simulink model "sara_restored_from_autosave"  (R2016a)
settings: Solver=VariableStepAuto  StartTime=0.0  StopTime=10  RelTol=1e-3
values from neighbouring files (symbols this model uses):
  s = a(1)*(t.^3)+a(2)*(t.^2)+a(3)*t+a(4)    [quydao.m]
undefined symbols (not defined in the file or in its folder): gia, k1, k2, k3, k4, RootGround, RootPart, sara
libraries: mblibv1 x17, simulink x1
settings Model: Creator=Admin  LastModifiedBy=Admin
settings GRTTargetCC: GeneratePreprocessorConditionals=Use local settings
settings SimMechanicsCC: VisOnUpdateDiagram=on  VisDuringSimulation=on

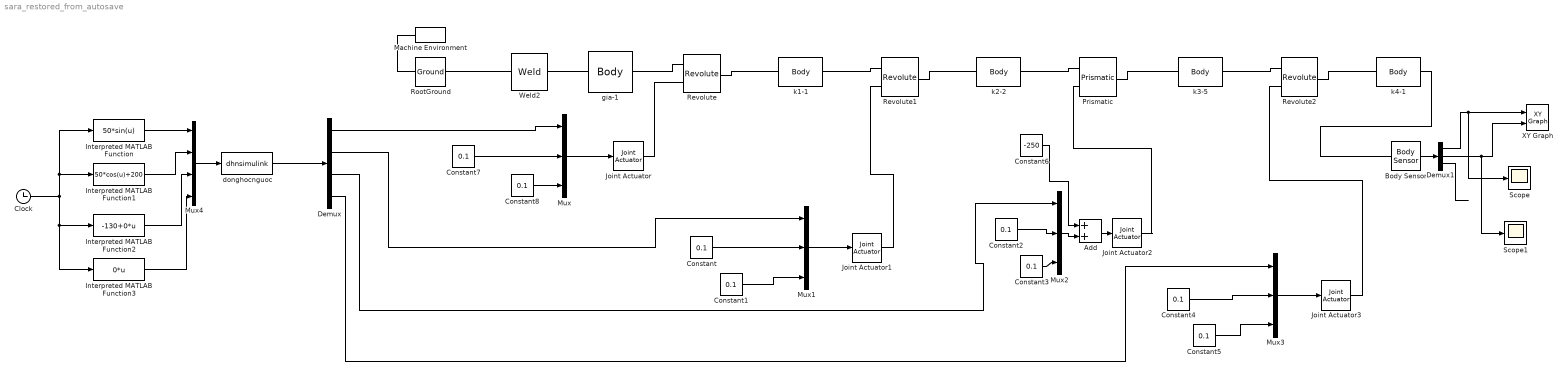
== system sara_restored_from_autosave ==
  Add : Sum
  Body Sensor : mblibv1/Sensors &  Actuators/Body Sensor  UpdateFromCAD=off  PhysicalDomain=Mechanical  PortType=blob  Muxed=on  Pose=off  Angle=on  AngleUnits=deg  ArcVelocity=off  ArcVelocityUnits=deg/s  ArcAcceleration=off  ArcAccelerationUnits=deg/s^2  CoordPosition=on  CoordPositionUnits=mm  Velocity=off  VelocityUnits=m/s  Acceleration=off  AccelerationUnits=m/s^2  Quaternion=on  QuaternionDT=off  QuaternionDDT=off  QuaternionUnits=off  OutputVector=[1]  ActiveIO=on  Width=3  DialogClass=MechanicalSensorBlock  ReferenceFrame=Absolute (World)
  Clock : Clock
  Constant{,1..5,7..8} (8 alike) : Constant  Value=0.1
  Constant6 : Constant  Value=-250
  Demux : Demux
  Demux1 : Demux  Outputs=3
  Interpreted MATLAB Function : MATLABFcn  MATLABFcn=50*sin(u)
  Interpreted MATLAB Function1 : MATLABFcn  MATLABFcn=50*cos(u)+200
  Interpreted MATLAB Function2 : MATLABFcn  MATLABFcn=-130+0*u
  Interpreted MATLAB Function3 : MATLABFcn  MATLABFcn=0*u
  Joint Actuator : mblibv1/Sensors &  Actuators/Joint Actuator  UpdateFromCAD=off  PhysicalDomain=Mechanical  PortType=blob  ActuationStyle=Motion  AngleUnits=rad  ArcVelocityUnits=rad/s  ArcAccelerationUnits=rad/s^2  CoordPositionUnits=m  VelocityUnits=m/s  AccelerationUnits=m/s^2  ForceUnits=N  TorqueUnits=N*m  ActiveIO=on  Width=3  DialogClass=MechanicalActuatorBlock  Primitive=R1  ReferenceFrame=Absolute (World)
  Joint Actuator1 : mblibv1/Sensors &  Actuators/Joint Actuator  UpdateFromCAD=off  PhysicalDomain=Mechanical  PortType=blob  ActuationStyle=Motion  AngleUnits=rad  ArcVelocityUnits=rad/s  ArcAccelerationUnits=rad/s^2  CoordPositionUnits=m  VelocityUnits=m/s  AccelerationUnits=m/s^2  ForceUnits=N  TorqueUnits=N*m  ActiveIO=on  Width=3  DialogClass=MechanicalActuatorBlock  Primitive=R1  ReferenceFrame=Absolute (World)
  Joint Actuator2 : mblibv1/Sensors &  Actuators/Joint Actuator  UpdateFromCAD=off  PhysicalDomain=Mechanical  PortType=blob  ActuationStyle=Motion  AngleUnits=deg  ArcVelocityUnits=deg/s  ArcAccelerationUnits=deg/s^2  CoordPositionUnits=mm  VelocityUnits=mm/s  AccelerationUnits=mm/s^2  ForceUnits=N  TorqueUnits=N*m  ActiveIO=on  Width=3  DialogClass=MechanicalActuatorBlock  Primitive=P1  ReferenceFrame=Absolute (World)
  Joint Actuator3 : mblibv1/Sensors &  Actuators/Joint Actuator  UpdateFromCAD=off  PhysicalDomain=Mechanical  PortType=blob  ActuationStyle=Motion  AngleUnits=rad  ArcVelocityUnits=rad/s  ArcAccelerationUnits=rad/s^2  CoordPositionUnits=m  VelocityUnits=m/s  AccelerationUnits=m/s^2  ForceUnits=N  TorqueUnits=N*m  ActiveIO=on  Width=3  DialogClass=MechanicalActuatorBlock  Primitive=R1  ReferenceFrame=Absolute (World)
  Machine Environment : mblibv1/Bodies/Machine Environment  PortType=env  PhysicalDomain=Mechanical  DialogTemplateClass=MECH.MachineEnvironment  SyncWhenCopied=off  Gravity="[0  0 -9.81]"  GravityUnits=m/s^2  GravityAsSignal=off  Dimensionality=Auto-detect  AnalysisType=Forward dynamics  LinearAssemblyTolerance=1e-3  LinearAssemblyToleranceUnits=m  AngularAssemblyTolerance=1e-3  AngularAssemblyToleranceUnits=rad  ConstraintSolverType=Stabilizing  ConstraintRelTolerance=1e-4  ConstraintAbsTolerance=1e-4  UseRobustSingularityHandling=off  RedundancyAnalysisToleranceType=Automatically select tolerance  RedundancyAnalysisTolerance=1e-14  StatePerturbationType=Fixed  PerturbationSize=1e-5  VisualizeMachine=on  BodyVisualizationType=Use model default body geometries  BodyColorSelMode=Use model default  DefaultBodyColor=[1 0 0]
  Mux{,1..3} (4 alike) : Mux  Inputs=3
  Mux4 : Mux
  Prismatic : mblibv1/Joints/Prismatic  LConnTagsString=__newl0|SA1  RConnTagsString=__newr0  UpdateFromCAD=on  PMImportedID=k2-2:-:k3-5  NumSAPorts=1  CutJoint=off  MarkAsCut=off  Primitives=prismatic  PrimitiveProps=P1$Base$[0,0,1]$prismatic  DialogClass=JointBlock  P1Axis=[0,0,1]
  Revolute : mblibv1/Joints/Revolute  LConnTagsString=__newl0|SA1  RConnTagsString=__newr0  UpdateFromCAD=on  PMImportedID=gia-1:-:k1-1  NumSAPorts=1  CutJoint=off  MarkAsCut=off  Primitives=prismatic  PrimitiveProps=R1$World$[0,0,1]$revolute  DialogClass=JointBlock  R1Axis=[0,0,1]
  Revolute1 : mblibv1/Joints/Revolute  LConnTagsString=__newl0|SA1  RConnTagsString=__newr0  UpdateFromCAD=on  PMImportedID=k1-1:-:k2-2  NumSAPorts=1  CutJoint=off  MarkAsCut=off  Primitives=prismatic  PrimitiveProps=R1$Base$[0,0,1]$revolute  DialogClass=JointBlock  R1Axis=[0,0,1]
  Revolute2 : mblibv1/Joints/Revolute  LConnTagsString=__newl0|SA1  RConnTagsString=__newr0  UpdateFromCAD=on  PMImportedID=k3-5:-:k4-1  NumSAPorts=1  CutJoint=off  MarkAsCut=off  Primitives=prismatic  PrimitiveProps=R1$Base$[0,0,1]$revolute  DialogClass=JointBlock  R1Axis=[0,0,1]
  RootGround : mblibv1/Bodies/Ground  UpdateFromCAD=on  PMImportedID=RootGround  LeftPortType=env  RightPortType=workingframe  PhysicalDomain=Mechanical  DialogClass=GroundBlock  CoordPosition=[0 0 0]  CoordPositionUnits=m  StateVectorMgrId=2  MachineId=[3 0]  ShowEnvPort=on  ParameterChecksum=[2920741816, 117602206, 132681718, 3781973339]  TopologyChecksum=[4066169678, 1305950860, 3136163654, 3539412486]
  Scope : Scope
  Scope1 : Scope
  Weld2 : mblibv1/Joints/Weld  LConnTagsString=__newl0  RConnTagsString=__newr0  UpdateFromCAD=on  PMImportedID=RootGround:-:sara/RootPart  NumSAPorts=0  CutJoint=off  MarkAsCut=off  Primitives=weld  PrimitiveProps=W$WORLD$[0.57735,0.57735,0.57735]$weld  DialogClass=JointBlock  WAxis=[0.57735,0.57735,0.57735]
  XY Graph : simulink/Sinks/XY Graph  xmin=-150  xmax=350  ymin=-100  ymax=300  st=-1
  donghocnguoc : MATLABFcn  MATLABFcn=dhnsimulink  OutputDimensions=4
  gia-1 : mblibv1/Bodies/Body  LConnTagsString=CS2  RConnTagsString=CS3  UpdateFromCAD=on  PMImportedID=gia-1  DialogClass=MechanicalBodyBlock  Mass=0.736659  MassUnits=kg  InertiaUnits=kg*m^2  Inertia=[0.0144639,0,0;0,0.0144639,0;0,0,0.000297178]  Shape=Cylinder  ShapeDims=[1 1]  ShapeUnits=m  ShapeUse=false  Density=1  DensityUnits=kg/m^3  DensityUse=false  GraphicsMode=GFXFILE  GraphicsFileName=sara - gia-1.STL  BodyColorSelMode=COLORPALETTE  BodyColor=[0.098039 0.79216 1]  AttachedToCS=CS1  CG=Right$CG$[0 0 -0.277667]$WORLD$WORLD$m$[1 0 0;0 1 0;0 0 1]$3x3 Transform$rad$WORLD$false$gia-1::CG(AUTOGEN)  WorkingFrames=Right$CS1$[0 0 -0.4]$WORLD$WORLD$m$[1 0 0;0 1 0;0 0 1]$3x3 Transform$rad$WORLD$false$gia-1::CS1(AUTOGEN)#Left$CS2$[0 0 0]$WORLD$WORLD$m$[1 0 0;0 1 0;0 0 1]$3x3 Transform$rad$WORLD$true$gia-1:-:sara/RootPart::gia-1(AUTOGEN)#Right$CS3$[0 0 0]$WORLD$WORLD$m$[1 0 0;0 1 0;0 0 1]$3x3 Transform$rad$WORLD$true$gia-1:-:k1-1::gia-1(AUTOGEN)#Right$CS4$[0 0 -0.4]$WORLD$WORLD$m$[1 0 0;0 1 0;0 0 1]$3x3 Transform$rad$WORLD$false$:-:sara/RootPart::gia-1(AUTOGEN)  CGPos=[0 0 -0.277667]  CGRot=[1 0 0;0 1 0;0 0 1]  CS0Pos=[]  CS0Rot=[]  CS1Pos=[0 0 -0.4]  CS1Rot=[1 0 0;0 1 0;0 0 1]  CS2Pos=[0 0 0]  CS2Rot=[1 0 0;0 1 0;0 0 1]  CS3Pos=[0 0 0]  CS3Rot=[1 0 0;0 1 0;0 0 1]  CS4Pos=[0 0 -0.4]  CS4Rot=[1 0 0;0 1 0;0 0 1]  CS5Pos=[]  CS5Rot=[]  CS6Pos=[]  CS6Rot=[]  CS7Pos=[]  CS7Rot=[]  CS8Pos=[]  CS8Rot=[]  CS9Pos=[]  CS9Rot=[]  CS10Pos=[]  CS10Rot=[]  CS11Pos=[]  CS11Rot=[]  CS12Pos=[]  CS12Rot=[]  CS13Pos=[]  CS13Rot=[]  CS14Pos=[]  CS14Rot=[]  CS15Pos=[]  CS15Rot=[]  CS16Pos=[]  CS16Rot=[]  CS17Pos=[]  CS17Rot=[]  CS18Pos=[]  CS18Rot=[]  CS19Pos=[]  CS19Rot=[]  CS20Pos=[]  CS20Rot=[]
  k1-1 : mblibv1/Bodies/Body  LConnTagsString=CS2  RConnTagsString=CS3  UpdateFromCAD=on  PMImportedID=k1-1  DialogClass=MechanicalBodyBlock  Mass=0.181133  MassUnits=kg  InertiaUnits=kg*m^2  Inertia=[3.45645e-05,0,-2.32643e-05;0,0.000746651,0;-2.32643e-05,0,0.000758713]  Shape=Cylinder  ShapeDims=[1 1]  ShapeUnits=m  ShapeUse=false  Density=1  DensityUnits=kg/m^3  DensityUse=false  GraphicsMode=GFXFILE  GraphicsFileName=sara - k1-1.STL  BodyColorSelMode=COLORPALETTE  BodyColor=[1;1;0]  AttachedToCS=CS1  CG=Right$CG$[0.112719 0 -0.00843903]$WORLD$WORLD$m$[1 0 0;0 1 0;0 0 1]$3x3 Transform$rad$WORLD$false$k1-1::CG(AUTOGEN)  WorkingFrames=Right$CS1$[0.0975 0 -0.02]$WORLD$WORLD$m$[1 0 0;0 1 0;0 0 1]$3x3 Transform$rad$WORLD$false$k1-1::CS1(AUTOGEN)#Left$CS2$[0 0 0]$WORLD$WORLD$m$[1 0 0;0 1 0;0 0 1]$3x3 Transform$rad$WORLD$true$gia-1:-:k1-1::k1-1(AUTOGEN)#Right$CS3$[0.195 0 0]$WORLD$WORLD$m$[1 0 0;0 1 0;0 0 1]$3x3 Transform$rad$WORLD$true$k1-1:-:k2-2::k1-1(AUTOGEN)  CGPos=[0.112719 0 -0.00843903]  CGRot=[1 0 0;0 1 0;0 0 1]  CS0Pos=[]  CS0Rot=[]  CS1Pos=[0.0975 0 -0.02]  CS1Rot=[1 0 0;0 1 0;0 0 1]  CS2Pos=[0 0 0]  CS2Rot=[1 0 0;0 1 0;0 0 1]  CS3Pos=[0.195 0 0]  CS3Rot=[1 0 0;0 1 0;0 0 1]  CS4Pos=[]  CS4Rot=[]  CS5Pos=[]  CS5Rot=[]  CS6Pos=[]  CS6Rot=[]  CS7Pos=[]  CS7Rot=[]  CS8Pos=[]  CS8Rot=[]  CS9Pos=[]  CS9Rot=[]  CS10Pos=[]  CS10Rot=[]  CS11Pos=[]  CS11Rot=[]  CS12Pos=[]  CS12Rot=[]  CS13Pos=[]  CS13Rot=[]  CS14Pos=[]  CS14Rot=[]  CS15Pos=[]  CS15Rot=[]  CS16Pos=[]  CS16Rot=[]  CS17Pos=[]  CS17Rot=[]  CS18Pos=[]  CS18Rot=[]  CS19Pos=[]  CS19Rot=[]  CS20Pos=[]  CS20Rot=[]
  k2-2 : mblibv1/Bodies/Body  LConnTagsString=CS2  RConnTagsString=CS3  UpdateFromCAD=on  PMImportedID=k2-2  DialogClass=MechanicalBodyBlock  Mass=0.0924482  MassUnits=kg  InertiaUnits=kg*m^2  Inertia=[1.24835e-05,0,0;0,0.000206205,0;0,0,0.00021007]  Shape=Cylinder  ShapeDims=[1 1]  ShapeUnits=m  ShapeUse=false  Density=1  DensityUnits=kg/m^3  DensityUse=false  GraphicsMode=GFXFILE  GraphicsFileName=sara - k2-2.STL  BodyColorSelMode=COLORPALETTE  BodyColor=[1;0;0]  AttachedToCS=CS1  CG=Right$CG$[0.270824 0 0.01]$WORLD$WORLD$m$[1 0 0;0 1 0;0 0 1]$3x3 Transform$rad$WORLD$false$k2-2::CG(AUTOGEN)  WorkingFrames=Right$CS1$[0.2675 0 0]$WORLD$WORLD$m$[1 0 0;0 1 0;0 0 1]$3x3 Transform$rad$WORLD$false$k2-2::CS1(AUTOGEN)#Left$CS2$[0.195 0 0]$WORLD$WORLD$m$[1 0 0;0 1 0;0 0 1]$3x3 Transform$rad$WORLD$true$k1-1:-:k2-2::k2-2(AUTOGEN)#Right$CS3$[0.34 0 0]$WORLD$WORLD$m$[1 0 0;0 -1 0;0 0 -1]$3x3 Transform$rad$CS1$true$k2-2:-:k3-5::k2-2(AUTOGEN)  CGPos=[0.270824 0 0.01]  CGRot=[1 0 0;0 1 0;0 0 1]  CS0Pos=[]  CS0Rot=[]  CS1Pos=[0.2675 0 0]  CS1Rot=[1 0 0;0 1 0;0 0 1]  CS2Pos=[0.195 0 0]  CS2Rot=[1 0 0;0 1 0;0 0 1]  CS3Pos=[0.34 0 0]  CS3Rot=[1 0 0;0 -1 0;0 0 -1]  CS4Pos=[]  CS4Rot=[]  CS5Pos=[]  CS5Rot=[]  CS6Pos=[]  CS6Rot=[]  CS7Pos=[]  CS7Rot=[]  CS8Pos=[]  CS8Rot=[]  CS9Pos=[]  CS9Rot=[]  CS10Pos=[]  CS10Rot=[]  CS11Pos=[]  CS11Rot=[]  CS12Pos=[]  CS12Rot=[]  CS13Pos=[]  CS13Rot=[]  CS14Pos=[]  CS14Rot=[]  CS15Pos=[]  CS15Rot=[]  CS16Pos=[]  CS16Rot=[]  CS17Pos=[]  CS17Rot=[]  CS18Pos=[]  CS18Rot=[]  CS19Pos=[]  CS19Rot=[]  CS20Pos=[]  CS20Rot=[]
  k3-5 : mblibv1/Bodies/Body  LConnTagsString=CS2  RConnTagsString=CS3  UpdateFromCAD=on  PMImportedID=k3-5  DialogClass=MechanicalBodyBlock  Mass=0.140347  MassUnits=kg  InertiaUnits=kg*m^2  Inertia=[0.00129427,0,0;0,1.27501e-05,0;0,0,0.00129427]  Shape=Cylinder  ShapeDims=[1 1]  ShapeUnits=m  ShapeUse=false  Density=1  DensityUnits=kg/m^3  DensityUse=false  GraphicsMode=GFXFILE  GraphicsFileName=sara - k3-5.STL  BodyColorSelMode=COLORPALETTE  BodyColor=[0;1;0]  AttachedToCS=CS1  CG=Right$CG$[0.34 0 -0.0864599]$WORLD$WORLD$m$[1 0 0;0 0 -1;0 1 0]$3x3 Transform$rad$WORLD$false$k3-5::CG(AUTOGEN)  WorkingFrames=Right$CS1$[0.34 0 0.03]$WORLD$WORLD$m$[1 0 0;0 0 -1;0 1 0]$3x3 Transform$rad$WORLD$false$k3-5::CS1(AUTOGEN)#Left$CS2$[0.34 0 0]$WORLD$WORLD$m$[1 0 0;0 1 0;0 0 1]$3x3 Transform$rad$WORLD$true$k2-2:-:k3-5::k3-5(AUTOGEN)#Right$CS3$[0.34 0 -0.25]$WORLD$WORLD$m$[1 0 0;0 -1 0;0 0 -1]$3x3 Transform$rad$WORLD$true$k3-5:-:k4-1::k3-5(AUTOGEN)  CGPos=[0.34 0 -0.0864599]  CGRot=[1 0 0;0 0 -1;0 1 0]  CS0Pos=[]  CS0Rot=[]  CS1Pos=[0.34 0 0.03]  CS1Rot=[1 0 0;0 0 -1;0 1 0]  CS2Pos=[0.34 0 0]  CS2Rot=[1 0 0;0 1 0;0 0 1]  CS3Pos=[0.34 0 -0.25]  CS3Rot=[1 0 0;0 -1 0;0 0 -1]  CS4Pos=[]  CS4Rot=[]  CS5Pos=[]  CS5Rot=[]  CS6Pos=[]  CS6Rot=[]  CS7Pos=[]  CS7Rot=[]  CS8Pos=[]  CS8Rot=[]  CS9Pos=[]  CS9Rot=[]  CS10Pos=[]  CS10Rot=[]  CS11Pos=[]  CS11Rot=[]  CS12Pos=[]  CS12Rot=[]  CS13Pos=[]  CS13Rot=[]  CS14Pos=[]  CS14Rot=[]  CS15Pos=[]  CS15Rot=[]  CS16Pos=[]  CS16Rot=[]  CS17Pos=[]  CS17Rot=[]  CS18Pos=[]  CS18Rot=[]  CS19Pos=[]  CS19Rot=[]  CS20Pos=[]  CS20Rot=[]
  k4-1 : mblibv1/Bodies/Body  LConnTagsString=CS3  RConnTagsString=CS2  UpdateFromCAD=on  PMImportedID=k4-1  DialogClass=MechanicalBodyBlock  Mass=0.0132102  MassUnits=kg  InertiaUnits=kg*m^2  Inertia=[2.70293e-05,0,0;0,2.71293e-05,0;0,0,2.77627e-07]  Shape=Cylinder  ShapeDims=[1 1]  ShapeUnits=m  ShapeUse=false  Density=1  DensityUnits=kg/m^3  DensityUse=false  GraphicsMode=GFXFILE  GraphicsFileName=sara - k4-1.STL  BodyColorSelMode=COLORPALETTE  BodyColor=[0;0;1]  AttachedToCS=CS1  CG=Right$CG$[0.34 0 -0.331654]$WORLD$WORLD$m$[0 -1 0;1 0 0;0 0 1]$3x3 Transform$rad$WORLD$false$k4-1::CG(AUTOGEN)  WorkingFrames=Right$CS1$[0.34 0 -0.38]$WORLD$WORLD$m$[0 -1 0;1 0 0;0 0 1]$3x3 Transform$rad$WORLD$false$k4-1::CS1(AUTOGEN)#Right$CS2$[0.34 0 -0.38]$WORLD$WORLD$m$[1 0 0;0 -1 0;0 0 -1]$3x3 Transform$rad$WORLD$true$k3-5:-:k4-1::k4-1(AUTOGEN)#Left$CS3$[0.34 0 -0.25]$WORLD$WORLD$m$[1 0 0;0 -1 0;0 0 -1]$3x3 Transform$rad$WORLD$true$none  CGPos=[0.34 0 -0.331654]  CGRot=[0 -1 0;1 0 0;0 0 1]  CS0Pos=[]  CS0Rot=[]  CS1Pos=[0.34 0 -0.38]  CS1Rot=[0 -1 0;1 0 0;0 0 1]  CS2Pos=[0.34 0 -0.38]  CS2Rot=[1 0 0;0 -1 0;0 0 -1]  CS3Pos=[0.34 0 -0.25]  CS3Rot=[1 0 0;0 -1 0;0 0 -1]  CS4Pos=[]  CS4Rot=[]  CS5Pos=[]  CS5Rot=[]  CS6Pos=[]  CS6Rot=[]  CS7Pos=[]  CS7Rot=[]  CS8Pos=[]  CS8Rot=[]  CS9Pos=[]  CS9Rot=[]  CS10Pos=[]  CS10Rot=[]  CS11Pos=[]  CS11Rot=[]  CS12Pos=[]  CS12Rot=[]  CS13Pos=[]  CS13Rot=[]  CS14Pos=[]  CS14Rot=[]  CS15Pos=[]  CS15Rot=[]  CS16Pos=[]  CS16Rot=[]  CS17Pos=[]  CS17Rot=[]  CS18Pos=[]  CS18Rot=[]  CS19Pos=[]  CS19Rot=[]  CS20Pos=[]  CS20Rot=[]
  wires:
  Mux/1 -> Joint Actuator/1
  Demux/1 -> Mux/1
  Constant7/1 -> Mux/2
  Constant8/1 -> Mux/3
  donghocnguoc/1 -> Demux/1
  Mux4/1 -> donghocnguoc/1
  Mux1/1 -> Joint Actuator1/1
  Demux/2 -> Mux1/1
  Constant/1 -> Mux1/2
  Constant1/1 -> Mux1/3
  Mux2/1 -> Add/2
  Demux/3 -> Mux2/1
  Constant2/1 -> Mux2/2
  Constant3/1 -> Mux2/3
  Mux3/1 -> Joint Actuator3/1
  Demux/4 -> Mux3/1
  Constant4/1 -> Mux3/2
  Constant5/1 -> Mux3/3
  Interpreted MATLAB Function/1 -> Mux4/1
  Interpreted MATLAB Function1/1 -> Mux4/2
  Interpreted MATLAB Function2/1 -> Mux4/3
  Interpreted MATLAB Function3/1 -> Mux4/4
  Clock/1 -> Interpreted MATLAB Function1/1, Interpreted MATLAB Function/1, Interpreted MATLAB Function3/1, Interpreted MATLAB Function2/1
  Add/1 -> Joint Actuator2/1
  Constant6/1 -> Add/1
  Body Sensor/1 -> Demux1/1
  Demux1/1 -> Scope/1, XY Graph/1
  Demux1/2 -> Scope1/1, XY Graph/2
  Demux1/3 -> ?
  connections:
  gia-1/RConn1 -- Revolute/LConn1
  Revolute/RConn1 -- k1-1/LConn1
  k1-1/RConn1 -- Revolute1/LConn1
  Revolute1/RConn1 -- k2-2/LConn1
  k2-2/RConn1 -- Prismatic/LConn1
  Prismatic/RConn1 -- k3-5/LConn1
  k3-5/RConn1 -- Revolute2/LConn1
  RootGround/RConn1 -- Weld2/LConn1
  RootGround/LConn1 -- Machine Environment/RConn1
  gia-1/LConn1 -- Weld2/RConn1
  Revolute2/RConn1 -- k4-1/LConn1
  Joint Actuator/RConn1 -- Revolute/LConn2
  Joint Actuator1/RConn1 -- Revolute1/LConn2
  Joint Actuator2/RConn1 -- Prismatic/LConn2
  Joint Actuator3/RConn1 -- Revolute2/LConn2
  k4-1/RConn1 -- Body Sensor/LConn1
